simulink model "power_KundurTwoAreaSystem"  (R2023a)
settings: Solver=FixedStepDiscrete  StartTime=0.0  StopTime=25  MaxStep=1/60  RelTol=1e-4
PreLoadFcn:
  | Ts=50e-6;
  | Tctrl=2*Ts;
  | PSSMODEL=1;
undefined symbols (not defined in the file): D1, Delta
libraries: spsGenericPowerSystemStabilizerLib x8, spsThreePhaseVIMeasurementLib x6, spsLoadFlowBusLib x6, spsThreePhaseParallelRLCLoadLib x4, spsThreePhasePISectionLineLib x4, spsSynchronousMachinepuStandardLib x4, spsExcitationSystemLib x4, spsSteamTurbineandGovernorLib x4, spsThreePhaseSeriesRLCLoadLib x4, spsThreePhaseTransformerTwoWindingsLib x4, spsThreePhaseBreakerLib x2, spsDistributedParametersLineLib x2
(part 2 of 2)

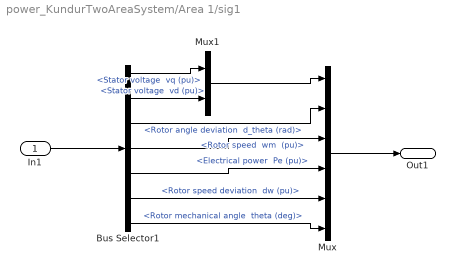
== system power_KundurTwoAreaSystem/Area 1/sig1 ==
  In1 : Inport
  Bus Selector1 : BusSelector  OutputSignals="dq0 components.Stator voltage  vq (pu),dq0 components.Stator voltage  vd (pu),Mechanical.Rotor angle deviation  d_theta (rad),Mechanical.Rotor speed  wm  (pu),Mechanical.Electrical power  Pe (pu),Mechanical.Rotor speed deviation  dw (pu),Mechanical.Rotor mechanical angle  theta (deg)"
  Mux : Mux  Inputs=6
  Mux1 : Mux  Inputs=2
  Out1 : Outport  VectorParamsAs1DForOutWhenUnconnected=off
  wires:
  Mux1/1 -> Mux/1
  Bus Selector1/1 -> Mux1/1  "<Stator voltage  vq (pu)>"
  Bus Selector1/2 -> Mux1/2  "<Stator voltage  vd (pu)>"
  Bus Selector1/3 -> Mux/2  "<Rotor angle deviation  d_theta (rad)>"
  Bus Selector1/4 -> Mux/3  "<Rotor speed  wm  (pu)>"
  Bus Selector1/5 -> Mux/4  "<Electrical power  Pe (pu)>"
  Bus Selector1/6 -> Mux/5  "<Rotor speed deviation  dw (pu)>"
  Bus Selector1/7 -> Mux/6  "<Rotor mechanical angle  theta (deg)>"
  In1/1 -> Bus Selector1/1
  Mux/1 -> Out1/1

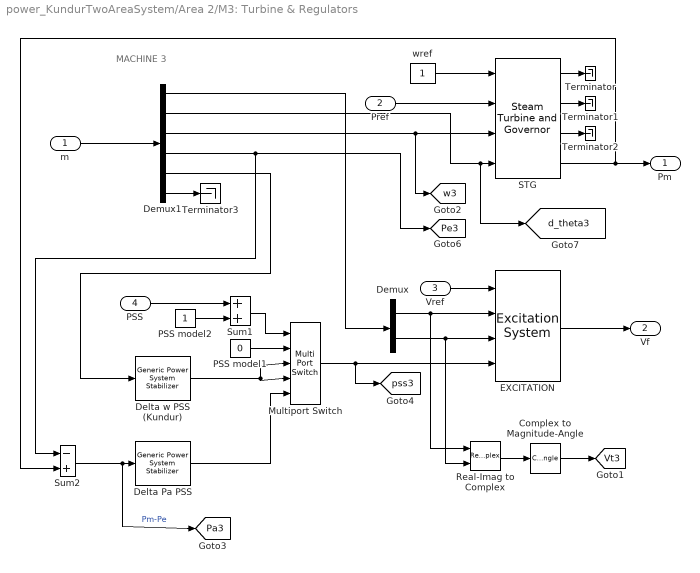
== system power_KundurTwoAreaSystem/Area 2/M3: Turbine & Regulators ==
  note: MACHINE 3
  m : Inport
  Pref : Inport  Port=2
  Vref : Inport  Port=3
  PSS : Inport  Port=4
  Complex to Magnitude-Angle : ComplexToMagnitudeAngle  Output=Magnitude
  Delta Pa PSS : spsGenericPowerSystemStabilizerLib/Generic Power System Stabilizer  Tsensor=15e-3  K=2.5*1.25  Twashout=1  Tleadlag1=[60e-3 1]  Tleadlag2=[0 0]  VSlimits=[-0.15 0.15]  Vinit=0  Plot_On=off  MagdB_On=on  FreqRange=logspace(-2,2,500)
      settings: LibrarySourceBlock=|
      | sps_lib/Electrical Machines/Synchronous Machine Control/Generic
      | Power System Stabilizer
  Delta w PSS (Kundur) : spsGenericPowerSystemStabilizerLib/Generic Power System Stabilizer  Tsensor=15e-3  K=30  Twashout=10  Tleadlag1=[50e-3 20e-3]  Tleadlag2=[3 5.4]  VSlimits=[-0.15 0.15]  Vinit=0  Plot_On=off  MagdB_On=on  FreqRange=logspace(-2,2,500)
      settings: LibrarySourceBlock=|
      | sps_lib/Electrical Machines/Synchronous Machine Control/Generic
      | Power System Stabilizer
  Demux : Demux  Outputs=2
      settings: DisplayOption=none
  Demux1 : Demux  Outputs=[2 1 1 1 1 1]
  EXCITATION : spsExcitationSystemLib/Excitation System  tr=20e-3  reg=[ 200, 0.001 ]  exc=[ 1, 0 ]  tgr=[ 0, 0 ]  damp=[ 0, 0 ]  sat=[ 0, 0 ]  lim=[ -12.3 , 12.3, 0 ]  v0=[1,1.83395]
      settings: LibrarySourceBlock=sps_lib/Electrical Machines/Synchronous Machine Control/Excitation System
  Multiport Switch : MultiPortSwitch  Inputs=4  SaturateOnIntegerOverflow=off
  PSS model1 : Constant  Value=0
  PSS model2 : Constant
  Real-Imag to Complex : RealImagToComplex
  STG : spsSteamTurbineandGovernorLib/Steam Turbine and Governor  gentype=Tandem-compound (single mass)  reg1="[ 1  0.05    0 ]"  reg2="[ 0.001  0.15 ]"  reg3="[ -0.1  0.1  0  4.496 ]"  N=3600  turb1="[ 0  10   3.3   0.5   ]"  turb2="[   0   0.36    0.36   0.28   ]"  HA="[ 0.046  1.430  1.465   0.192 ]"  KA="[ 90.44  53.88  64.59   62.94  ]"  DA="[ 0.0115  0.3575  0.3663   0.0137  ]"  ini1=0.798889  ini2=[0.800505,-56.3243]
      settings: LibrarySourceBlock=|
      | sps_lib/Electrical Machines/Synchronous Machine Control/Steam Turbine
      | and Governor
  Sum1 : Sum  InputSameDT=on  SaturateOnIntegerOverflow=on  OutDataTypeStr=Inherit: Same as first input
  Sum2 : Sum  Inputs=-+  InputSameDT=on  SaturateOnIntegerOverflow=on  OutDataTypeStr=Inherit: Same as first input
  Terminator{,1..3} (4 alike) : Terminator
  wref : Constant
  Pm : Outport  InitialOutput=0  VectorParamsAs1DForOutWhenUnconnected=off
  Vf : Outport  Port=2  InitialOutput=0  VectorParamsAs1DForOutWhenUnconnected=off
  tag scope: Pa3=global, Pe3=global, Vt3=global, d_theta3=global, pss3=global, w3=global
  wires:
  Sum2/1 -> [Pa3], Delta Pa PSS/1  "Pm-Pe"
  Demux1/5 -> Delta w PSS (Kundur)/1
  Demux1/4 -> Sum2/1, [Pe3]
  Demux1/3 -> [w3], STG/3
  Demux1/1 -> Demux/1
  PSS/1 -> Sum1/1
  Sum1/1 -> Multiport Switch/1
  PSS model2/1 -> Sum1/2
  Delta Pa PSS/1 -> Multiport Switch/5
  Delta w PSS (Kundur)/1 -> Multiport Switch/4, Multiport Switch/3
  PSS model1/1 -> Multiport Switch/2
  Multiport Switch/1 -> [pss3], EXCITATION/4
  Demux1/6 -> Terminator3/1
  Complex to Magnitude-Angle/1 -> [Vt3]
  EXCITATION/1 -> Vf/1
  Real-Imag to Complex/1 -> Complex to Magnitude-Angle/1
  Vref/1 -> EXCITATION/1
  m/1 -> Demux1/1
  Pref/1 -> STG/2
  wref/1 -> STG/1
  Demux/2 -> Real-Imag to Complex/2, EXCITATION/3
  Demux/1 -> Real-Imag to Complex/1, EXCITATION/2
  Demux1/2 -> [d_theta3], STG/4
  STG/1 -> Terminator/1
  STG/2 -> Terminator1/1
  STG/3 -> Terminator2/1
  STG/4 -> Pm/1, Sum2/2

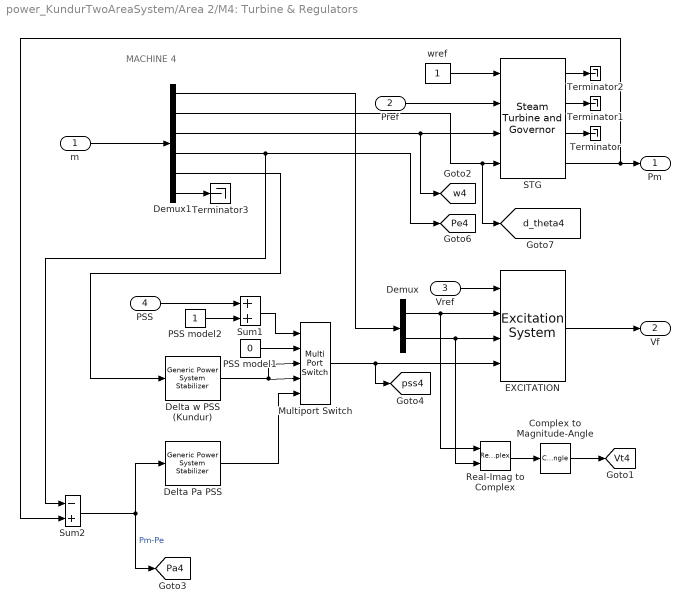
== system power_KundurTwoAreaSystem/Area 2/M4: Turbine & Regulators ==
  note: MACHINE 4
  m : Inport
  Pref : Inport  Port=2
  Vref : Inport  Port=3
  PSS : Inport  Port=4
  Complex to Magnitude-Angle : ComplexToMagnitudeAngle  Output=Magnitude
  "Delta Pa PSS " : spsGenericPowerSystemStabilizerLib/Generic Power System Stabilizer  Tsensor=15e-3  K=2.5*1.25  Twashout=1  Tleadlag1=[60e-3 1]  Tleadlag2=[0 0]  VSlimits=[-0.15 0.15]  Vinit=0  Plot_On=off  MagdB_On=on  FreqRange=logspace(-2,2,500)
      settings: LibrarySourceBlock=|
      | sps_lib/Electrical Machines/Synchronous Machine Control/Generic
      | Power System Stabilizer
  Delta w PSS (Kundur) : spsGenericPowerSystemStabilizerLib/Generic Power System Stabilizer  Tsensor=15e-3  K=30  Twashout=10  Tleadlag1=[50e-3 20e-3]  Tleadlag2=[3 5.4]  VSlimits=[-0.15 0.15]  Vinit=0  Plot_On=off  MagdB_On=on  FreqRange=logspace(-2,2,500)
      settings: LibrarySourceBlock=|
      | sps_lib/Electrical Machines/Synchronous Machine Control/Generic
      | Power System Stabilizer
  Demux : Demux  Outputs=2
      settings: DisplayOption=none
  Demux1 : Demux  Outputs=[2 1 1 1 1 1]
  EXCITATION : spsExcitationSystemLib/Excitation System  tr=20e-3  reg=[ 200, 0.001 ]  exc=[ 1, 0 ]  tgr=[ 0, 0 ]  damp=[ 0, 0 ]  sat=[ 0, 0 ]  lim=[ -12.3 , 12.3, 0 ]  v0=[1,1.83395]
      settings: LibrarySourceBlock=sps_lib/Electrical Machines/Synchronous Machine Control/Excitation System
  Multiport Switch : MultiPortSwitch  Inputs=4  SaturateOnIntegerOverflow=off
  PSS model1 : Constant  Value=0
  PSS model2 : Constant
  Real-Imag to Complex : RealImagToComplex
  STG : spsSteamTurbineandGovernorLib/Steam Turbine and Governor  gentype=Tandem-compound (single mass)  reg1="[ 1  0.05    0 ]"  reg2="[ 0.001  0.15 ]"  reg3="[ -0.1  0.1  0  4.496 ]"  N=3600  turb1="[ 0  10   3.3   0.5   ]"  turb2="[   0   0.36    0.36   0.28   ]"  HA="[ 0.046  1.430  1.465   0.192 ]"  KA="[ 90.44  53.88  64.59   62.94  ]"  DA="[ 0.0115  0.3575  0.3663   0.0137  ]"  ini1=0.7778  ini2=[0.779311,-67.7513]
      settings: LibrarySourceBlock=|
      | sps_lib/Electrical Machines/Synchronous Machine Control/Steam Turbine
      | and Governor
  Sum1 : Sum  InputSameDT=on  SaturateOnIntegerOverflow=on  OutDataTypeStr=Inherit: Same as first input
  Sum2 : Sum  Inputs=-+  InputSameDT=on  SaturateOnIntegerOverflow=on  OutDataTypeStr=Inherit: Same as first input
  Terminator{,1..3} (4 alike) : Terminator
  wref : Constant
  Pm : Outport  InitialOutput=0  VectorParamsAs1DForOutWhenUnconnected=off
  Vf : Outport  Port=2  InitialOutput=0  VectorParamsAs1DForOutWhenUnconnected=off
  tag scope: Pa4=global, Pe4=global, Vt4=global, d_theta4=global, pss4=global, w4=global
  wires:
  Demux/1 -> Real-Imag to Complex/1, EXCITATION/2
  Demux/2 -> Real-Imag to Complex/2, EXCITATION/3
  STG/4 -> Pm/1, Sum2/2
  wref/1 -> STG/1
  Pref/1 -> STG/2
  m/1 -> Demux1/1
  Vref/1 -> EXCITATION/1
  STG/3 -> Terminator/1
  Real-Imag to Complex/1 -> Complex to Magnitude-Angle/1
  EXCITATION/1 -> Vf/1
  Complex to Magnitude-Angle/1 -> [Vt4]
  Demux1/6 -> Terminator3/1
  Multiport Switch/1 -> EXCITATION/4, [pss4]
  PSS model1/1 -> Multiport Switch/2
  Delta w PSS (Kundur)/1 -> Multiport Switch/4, Multiport Switch/3
  "Delta Pa PSS "/1 -> Multiport Switch/5
  PSS model2/1 -> Sum1/2
  Sum1/1 -> Multiport Switch/1
  PSS/1 -> Sum1/1
  Demux1/1 -> Demux/1
  Demux1/3 -> [w4], STG/3
  Demux1/4 -> Sum2/1, [Pe4]
  Demux1/5 -> Delta w PSS (Kundur)/1
  Sum2/1 -> "Delta Pa PSS "/1, [Pa4]  "Pm-Pe"
  STG/2 -> Terminator1/1
  STG/1 -> Terminator2/1
  Demux1/2 -> [d_theta4], STG/4

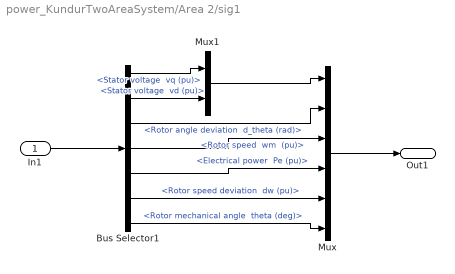
== system power_KundurTwoAreaSystem/Area 2/sig1 ==
  In1 : Inport
  Bus Selector1 : BusSelector  OutputSignals="dq0 components.Stator voltage  vq (pu),dq0 components.Stator voltage  vd (pu),Mechanical.Rotor angle deviation  d_theta (rad),Mechanical.Rotor speed  wm  (pu),Mechanical.Electrical power  Pe (pu),Mechanical.Rotor speed deviation  dw (pu),Mechanical.Rotor mechanical angle  theta (deg)"
  Mux : Mux  Inputs=6
  Mux1 : Mux  Inputs=2
  Out1 : Outport  VectorParamsAs1DForOutWhenUnconnected=off
  wires:
  Mux1/1 -> Mux/1
  Bus Selector1/1 -> Mux1/1  "<Stator voltage  vq (pu)>"
  Bus Selector1/2 -> Mux1/2  "<Stator voltage  vd (pu)>"
  Bus Selector1/3 -> Mux/2  "<Rotor angle deviation  d_theta (rad)>"
  Bus Selector1/4 -> Mux/3  "<Rotor speed  wm  (pu)>"
  Bus Selector1/5 -> Mux/4  "<Electrical power  Pe (pu)>"
  Bus Selector1/6 -> Mux/5  "<Rotor speed deviation  dw (pu)>"
  Bus Selector1/7 -> Mux/6  "<Rotor mechanical angle  theta (deg)>"
  In1/1 -> Bus Selector1/1
  Mux/1 -> Out1/1

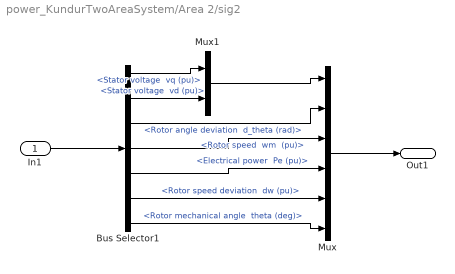
== system power_KundurTwoAreaSystem/Area 2/sig2 ==
  In1 : Inport
  Bus Selector1 : BusSelector  OutputSignals="dq0 components.Stator voltage  vq (pu),dq0 components.Stator voltage  vd (pu),Mechanical.Rotor angle deviation  d_theta (rad),Mechanical.Rotor speed  wm  (pu),Mechanical.Electrical power  Pe (pu),Mechanical.Rotor speed deviation  dw (pu),Mechanical.Rotor mechanical angle  theta (deg)"
  Mux : Mux  Inputs=6
  Mux1 : Mux  Inputs=2
  Out1 : Outport  VectorParamsAs1DForOutWhenUnconnected=off
  wires:
  Mux1/1 -> Mux/1
  Bus Selector1/1 -> Mux1/1  "<Stator voltage  vq (pu)>"
  Bus Selector1/2 -> Mux1/2  "<Stator voltage  vd (pu)>"
  Bus Selector1/3 -> Mux/2  "<Rotor angle deviation  d_theta (rad)>"
  Bus Selector1/4 -> Mux/3  "<Rotor speed  wm  (pu)>"
  Bus Selector1/5 -> Mux/4  "<Electrical power  Pe (pu)>"
  Bus Selector1/6 -> Mux/5  "<Rotor speed deviation  dw (pu)>"
  Bus Selector1/7 -> Mux/6  "<Rotor mechanical angle  theta (deg)>"
  In1/1 -> Bus Selector1/1
  Mux/1 -> Out1/1
